simulink model "Childs_Mobile"  (R2024a)
settings: Solver=FixedStepAuto  StartTime=0.0  StopTime=inf  RelTol=1e-3
libraries: androiduilib x6, androidcommunicationlib x4, androidaudiovideolib x3, androidsensorlib x2, fuzblock x1
settings Model: Creator=Omkar R Prabhu  LastModifiedBy=Omkar R Prabhu
settings OptimizationCC: EnhancedBackFolding=on  PassReuseOutputArgsAs=Individual arguments  ZeroExternalMemoryAtStartup=off  ZeroInternalMemoryAtStartup=off  MaxStackSize=64  OptimizeBlockOrder=speed  DifferentSizesBufferReuse=on  OptimizationCustomize=off  EfficientTunableParamExpr=on
settings DebuggingCC: ParameterTunabilityLossMsg=error
settings HardwareCC: ProdBitPerPointer=32  ProdBitPerSizeT=32  ProdBitPerPtrDiffT=32  ProdLargestAtomicInteger=Long  ProdLargestAtomicFloat=Double  ProdWordSize=32  ProdHWDeviceType=ARM Compatible->ARM Cortex  UseEmbeddedCoderFeatures=off  UseSimulinkCoderFeatures=off
settings SFSimCC: MATLABDynamicMemAlloc=off
settings RTWCC: Description=Embedded Coder  SystemTargetFile=ert.tlc  HardwareBoard=Android Device  TLCOptions="-aInlineSetEventsForThisBaseRateFcn=TLC_FALSE -aSuppressMultiTaskScheduler=TLC_FALSE  -aRateBasedStepFcn=0"  TemplateMakefile=ert_default_tmf  RTWVerbose=off  Toolchain=Android SDK/NDK Tools
settings CodeAppCC: ForceParamTrailComments=on  IgnoreCustomStorageClasses=off  OperatorAnnotations=on  SimulinkDataObjDesc=on  SFDataObjDesc=on  InsertBlockDesc=on
settings ERTTargetCC: SupportNonInlinedSFcns=on

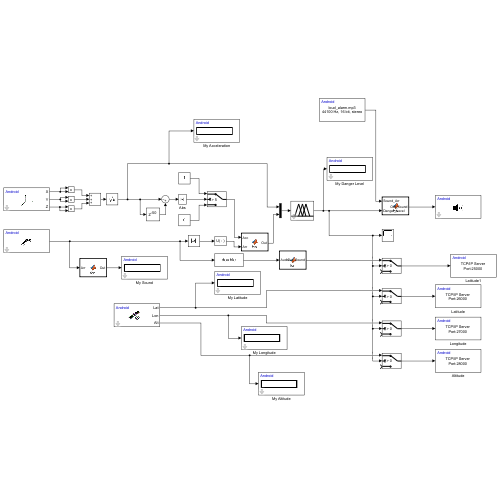
[thumbnail: Simulink's stored preview of the top-level diagram]
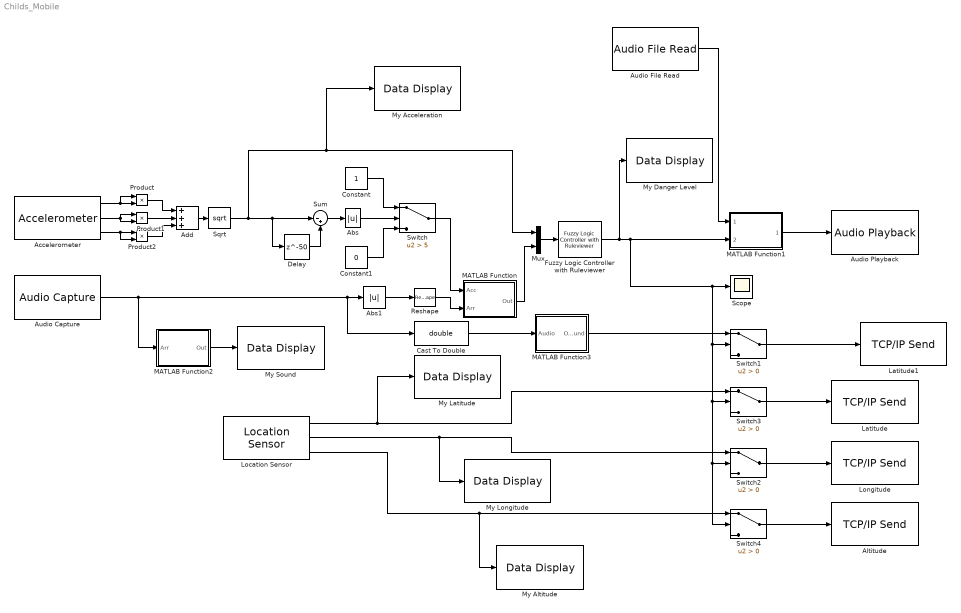
== system Childs_Mobile ==
  Abs : Abs  SaturateOnIntegerOverflow=off
  Abs1 : Abs  SaturateOnIntegerOverflow=off
  Accelerometer : androidsensorlib/Accelerometer  OutputVector=off  SampleTime=0.1  BlockPlatform=Android
  Add : Sum  Inputs=+++
  Altitude : androidcommunicationlib/TCP//IP Send  TCPSendId=Childs_Mobile/Altitude  Mode_=Server  LocalServerPort_=28000  RemoteAddr_=127.0.0.4  RemoteServerPort_=25000  ClientPortBindingSelection_=off  ClientPortToBind_=35000  BlockingMode_=off  BlockTimeout_=0.1
  Audio Capture : androidaudiovideolib/Audio Capture  SampleFreq=44100  FrameSize=4410  SampleTime=0.1  SimulateUsing=Code generation  DeviceStr=0  QueueDuration=0  BlockPlatform=Android  AudioSamplingFreq=44100
  Audio File Read : androidaudiovideolib/Audio File Read  FileName=C:\Users\OmkarRPrabhu\OneDrive - iitgn.ac.in\Desktop\Assignments\loud_alarm.mp3  FrameSize=4410
  Audio Playback : androidaudiovideolib/Audio Playback  SampleFreq=44100  AudioSamplingFreq=44100  SampleTime=0.1  DeviceStr=0  QueueDuration=0  BlockPlatform=Android
  Cast To Double : DataTypeConversion  OutDataTypeStr=double  SaturateOnIntegerOverflow=off  RndMeth=Floor
  Constant : Constant
  Constant1 : Constant  Value=0
  Delay : Delay  DelayLength=50  InitialCondition=0
  Fuzzy Logic Controller with Ruleviewer : fuzblock/Fuzzy Logic  Controller  with Ruleviewer  fismatrix=mamdanitype1  Ts=2
  Latitude : androidcommunicationlib/TCP//IP Send  TCPSendId=Childs_Mobile/Latitude  Mode_=Server  LocalServerPort_=26000  RemoteAddr_=127.0.0.2  RemoteServerPort_=25000  ClientPortBindingSelection_=off  ClientPortToBind_=35000  BlockingMode_=off  BlockTimeout_=0.1
  Latitude1 : androidcommunicationlib/TCP//IP Send  TCPSendId=Childs_Mobile/Latitude1  Mode_=Server  LocalServerPort_=25000  RemoteAddr_=127.0.0.2  RemoteServerPort_=25000  ClientPortBindingSelection_=off  ClientPortToBind_=35000  BlockingMode_=off  BlockTimeout_=0.1
  Location Sensor : androidsensorlib/Location Sensor  OutputVector=off  SampleTime=0.1  BlockPlatform=Android
  Longitude : androidcommunicationlib/TCP//IP Send  TCPSendId=Childs_Mobile/Longitude  Mode_=Server  LocalServerPort_=27000  RemoteAddr_=127.0.0.3  RemoteServerPort_=25000  ClientPortBindingSelection_=off  ClientPortToBind_=35000  BlockingMode_=off  BlockTimeout_=0.1
  MATLAB Function : MATLAB Function  TreatAsAtomicUnit=on
  MATLAB Function1 : MATLAB Function  TreatAsAtomicUnit=on
  MATLAB Function2 : MATLAB Function  TreatAsAtomicUnit=on
  MATLAB Function3 : MATLAB Function  TreatAsAtomicUnit=on
  Mux : Mux  Inputs=2
  My Acceleration : androiduilib/Data Display  DataDisplayId=Childs_Mobile/My_Acceleration  Format=Float  Precision=6  SimulateUsing=Code generation  blockPlatform=Android
  My Altitude : androiduilib/Data Display  DataDisplayId=Childs_Mobile/My_Altitude  Format=Float  Precision=6  SimulateUsing=Code generation  blockPlatform=Android
  My Danger Level : androiduilib/Data Display  DataDisplayId=Childs_Mobile/My_Danger_Level  Format=Float  Precision=6  SimulateUsing=Code generation  blockPlatform=Android
  My Latitude : androiduilib/Data Display  DataDisplayId=Childs_Mobile/My_Latitude  Format=Float  Precision=6  SimulateUsing=Code generation  blockPlatform=Android
  My Longitude : androiduilib/Data Display  DataDisplayId=Childs_Mobile/My_Longitude  Format=Float  Precision=6  SimulateUsing=Code generation  blockPlatform=Android
  My Sound : androiduilib/Data Display  DataDisplayId=Childs_Mobile/My_Sound  Format=Float  Precision=6  SimulateUsing=Code generation  blockPlatform=Android
  Product : Product
  Product1 : Product
  Product2 : Product
  Reshape : Reshape
  Scope : Scope
  Sqrt : Sqrt
  Sum : Sum  Inputs=|-+
  Switch : Switch  Criteria=u2 > Threshold  Threshold=5  SaturateOnIntegerOverflow=off  InputSameDT=off
  Switch1 : Switch  Criteria=u2 > Threshold  OutDataTypeStr=int16  SaturateOnIntegerOverflow=off  InputSameDT=off
  Switch2 : Switch  Criteria=u2 > Threshold  SaturateOnIntegerOverflow=off  InputSameDT=off
  Switch3 : Switch  Criteria=u2 > Threshold  SaturateOnIntegerOverflow=off  InputSameDT=off
  Switch4 : Switch  Criteria=u2 > Threshold  SaturateOnIntegerOverflow=off  InputSameDT=off
  wires:
  Constant1/1 -> Switch/3
  MATLAB Function1/1(Out_Sound) -> Audio Playback/1
  Switch3/1 -> Latitude/1
  Switch2/1 -> Longitude/1
  Location Sensor/1 -> My Latitude/1, Switch3/1
  Audio File Read/1 -> MATLAB Function1/1(Sound_Arr)
  Mux/1 -> Fuzzy Logic Controller with Ruleviewer/1
  Abs1/1 -> Reshape/1
  Add/1 -> Sqrt/1
  Sqrt/1 -> Delay/1, Sum/1, My Acceleration/1, Mux/1
  Constant/1 -> Switch/1
  Reshape/1 -> MATLAB Function/2(Arr)
  MATLAB Function/1(Out) -> Mux/2
  Audio Capture/1 -> MATLAB Function2/1(Arr), Cast To Double/1, Abs1/1
  Product1/1 -> Add/2
  Product2/1 -> Add/3
  Accelerometer/1 -> Product/1, Product/2
  Product/1 -> Add/1
  Switch/1 -> MATLAB Function/1(Acc)
  Abs/1 -> Switch/2
  Accelerometer/2 -> Product1/1, Product1/2
  Location Sensor/2 -> My Longitude/1, Switch2/1
  Sum/1 -> Abs/1
  Delay/1 -> Sum/2
  Accelerometer/3 -> Product2/2, Product2/1
  Switch4/1 -> Altitude/1
  Location Sensor/3 -> My Altitude/1, Switch4/1
  Fuzzy Logic Controller with Ruleviewer/1 -> My Danger Level/1, Scope/1, Switch1/2, Switch3/2, Switch4/2, Switch2/2, MATLAB Function1/2(Danger_Level)
  MATLAB Function2/1(Out) -> My Sound/1
  Switch1/1 -> Latitude1/1
  Cast To Double/1 -> MATLAB Function3/1(Audio)
  MATLAB Function3/1(Out_Sound) -> Switch1/1

== matlab function Childs_Mobile/MATLAB Function1 ==
  data: Sound_Arr input; Danger_Level input; Out_Sound output
function Out_Sound = fcn(Sound_Arr , Danger_Level)
    if(Danger_Level <= 0.333333)
        Out_Sound = Sound_Arr.*0 ; 
    else if (Danger_Level <= 0.6666)
        Out_Sound = Sound_Arr.*0.1 ;
    else 
        Out_Sound = Sound_Arr ; 
        end
    end 
end

== matlab function Childs_Mobile/MATLAB Function2 ==
  data: Arr input; Out output
function Out = fcn(Arr)
    Out = single(max(Arr)) ; 
end

== matlab function Childs_Mobile/MATLAB Function3 ==
  data: Audio input; Out_Sound output
function Out_Sound = fcn(Audio)
    Out_Sound  = Audio(:,1) ;
end

== matlab function Childs_Mobile/MATLAB Function ==
  data: Acc input; Arr input; Out output
function Out = fcn(Acc , Arr)
    if(Acc == 1)
        Out = single(max(Arr)) ; 
    else 
        Out = single(0) ; 
    end 
end
